simulink model "ff_test"  (R2023b)
settings: Solver=VariableStepAuto  StartTime=0.0  StopTime=10  RelTol=1e-3
values from neighbouring files (symbols this model uses):
  D = 0.000001    (= 1e-06)    [motor_param.m]
  J = 0.151e-7    (= 1.51e-08)    [motor_param.m]
  K_e = 1    [ff_inv.m]    (also in motor_param.m = 0.00352372567731)
  K_t = 1    [ff_inv.m]    (also in motor_param.m = 0.00352)
  L = 0.045    [motor_param.m]
  m = 1    [ff_inv.m]    (also in motor_param.m = 0.15)
  r = 1    [ff_inv.m]    (also in motor_param.m = 0.012)
  R = 1    [ff_inv.m]    (also in motor_param.m = 2.9)
settings Model: Creator=under  LastModifiedBy=under

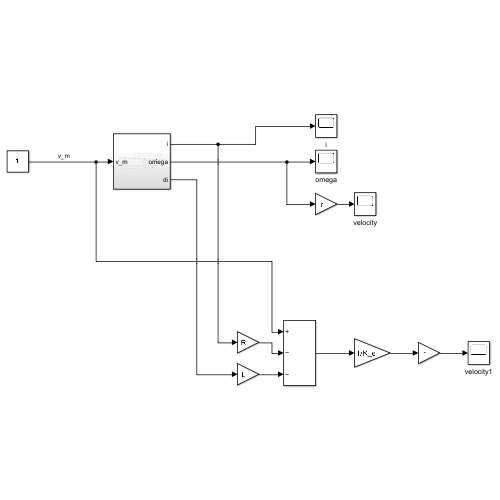
[thumbnail: Simulink's stored preview of the top-level diagram]
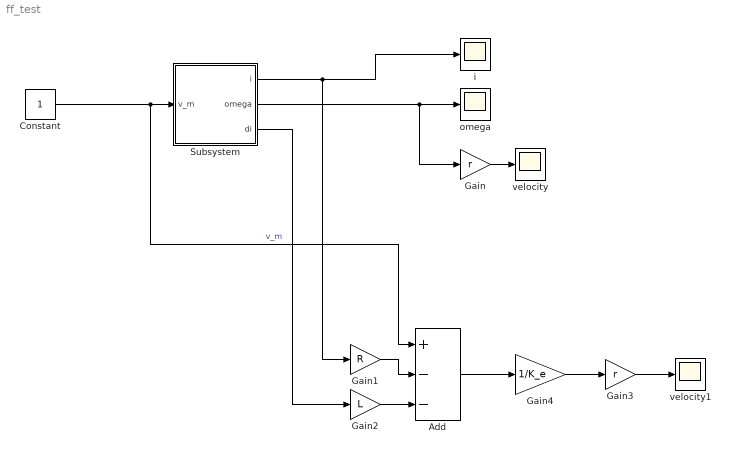
== system ff_test ==
  Add : Sum  Inputs=+--
  Constant : Constant
  Gain : Gain  Gain=r
  Gain1 : Gain  Gain=R
  Gain2 : Gain  Gain=L
  Gain3 : Gain  Gain=r
  Gain4 : Gain  Gain=1/K_e
  Subsystem : Subsystem
  i : Scope
  omega : Scope
  velocity : Scope
  velocity1 : Scope
  wires:
  Constant/1 -> Add/1, Subsystem/1(v_m)  "v_m"
  Subsystem/1(i) -> Gain1/1, i/1
  Subsystem/2(omega) -> Gain/1, omega/1
  Gain/1 -> velocity/1
  Gain1/1 -> Add/2
  Gain2/1 -> Add/3
  Subsystem/3(di) -> Gain2/1
  Add/1 -> Gain4/1
  Gain3/1 -> velocity1/1
  Gain4/1 -> Gain3/1

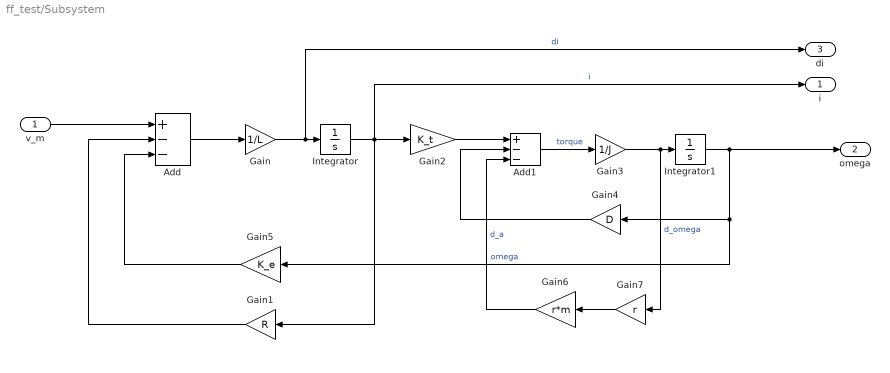
== system ff_test/Subsystem ==
  v_m : Inport
  Add : Sum  Inputs=+--
  Add1 : Sum  Inputs=+--
  Gain : Gain  Gain=1/L
  Gain1 : Gain  Gain=R
  Gain2 : Gain  Gain=K_t
  Gain3 : Gain  Gain=1/J
  Gain4 : Gain  Gain=D
  Gain5 : Gain  Gain=K_e
  Gain6 : Gain  Gain=r*m
  Gain7 : Gain  Gain=r
  Integrator : Integrator
  Integrator1 : Integrator
  i : Outport
  omega : Outport  Port=2
  di : Outport  Port=3
  wires:
  Gain5/1 -> Add/3
  Gain2/1 -> Add1/1
  Gain3/1 -> Gain7/1, Integrator1/1  "d_omega"
  Integrator/1 -> i/1, Gain2/1, Gain1/1  "i"
  Gain1/1 -> Add/2
  Gain/1 -> di/1, Integrator/1  "di"
  Add/1 -> Gain/1
  Integrator1/1 -> omega/1, Gain4/1, Gain5/1  "omega"
  Add1/1 -> Gain3/1  "torque"
  Gain4/1 -> Add1/2
  v_m/1 -> Add/1
  Gain6/1 -> Add1/3  "d_a"
  Gain7/1 -> Gain6/1
